simulink model "sim1"  (R2025a)
settings: Solver=VariableStepAuto  StartTime=0.0  StopTime=150  RelTol=1e-3
InitFcn:
  | clc;
  | close all;
  | clear;
  | s=tf('s');
  | G11=(0.806*s+0.264)/(s^2+1.15*s+0.202);
  | G12=-(15*s+1.42)/(s^3+12.8*s^2+13.6*s+2.36);
  | G21=(1.95*s^2+2.12*s+0.49)/(s^3+9.15*s^2+9.39*s+1.62);
  | G22=(7.14*s^2+25.8*s+9.35)/(s^4+20.8*s^3+116.4*s^2+111.6*s+18.8);
  | G=[G11,G12;G21,G22];
  | a11=[1 1.15 0.202];
  | a12=[1 12.8 13.6 2.36];
  | a21=[1 9.15 9.39 1.62];
  | a22=[1 20.8 116.4 111.6 18.8];
  | b11=[0.806 0.264];
  | b12=-[15 1.42];
  | b21=[1.95 2.12 0.49];
  | b22=[7.14 25.8 9.35];
  | K=[2,2.5;-6,5.5];
  | Q11=K(1,1)*G11+K(2,1)*G12;
  | Q12=K(1,2)*G11+K(2,2)*G12;
  | Q21=K(1,1)*G21+K(2,1)*G22;
  | Q22=K(1,2)*G21+K(2,2)*G22;
  | Q=[Q11,Q12;Q21,Q22];
  | % Gershgorinbands_MIMO(Q)
  | f1=1;
  | f2=1;
  | t11=(1/f1+Q11);
  | t12=(Q12);
  | t21=(Q21);
  | t22=(1/f2+Q22);
  | C1=pidtune(t11,'pi');
  | C2=pidtune(t22,'pi');
  | P1=C1.Kp;
  | I1=C1.Ki;
  | D1=C1.Kd;
  | P2=C2.Kp;
  | I2=C2.Ki;
  | D2=C2.Kd;
StopFcn:
  | close all;
  | subplot(1,2,1)
  | plot(out.tout,out.y_ref.data(:,1),'-.','LineWidth',3.5)
  | hold on
  | plot(out.tout,out.y.data(:,1),'LineWidth',2.5)
  | xlabel('time')
  | ylabel('y_1')
  | grid
  | subplot(1,2,2)
  | plot(out.tout,out.y_ref.data(:,2),'-.','LineWidth',3.5)
  | hold on
  | plot(out.tout,out.y.data(:,2),'LineWidth',2.5)
  | xlabel('time')
  | ylabel('y_2')
  | grid
  | sgtitle('System response')
  | 
  | figure()
  | subplot(1,2,1)
  | plot(out.tout,out.u.data(:,1),'LineWidth',2.5)
  | xlabel('time')
  | ylabel('u_1')
  | grid
  | subplot(1,2,2)
  | plot(out.tout,out.u.data(:,2),'LineWidth',2.5)
  | xlabel('time')
  | ylabel('u_2')
  | grid
  | sgtitle('Control Signal')
libraries: slpidlib x2, simulink x2
settings Model: Creator=rz97e  LastModifiedBy=sohrab
settings ModelReferenceCC: EnableRefExpFcnMdlSchedulingChecks=on
settings RTWCC: GPUComputeCapability=3.5

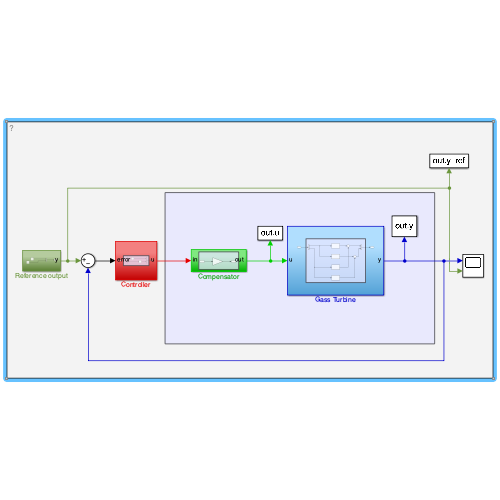
[thumbnail: Simulink's stored preview of the top-level diagram]
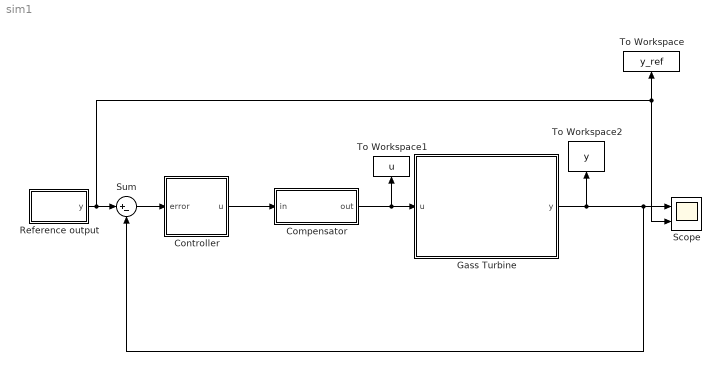
== system sim1 ==
  Compensator : Subsystem
  Controller : Subsystem
  Gass Turbine : Subsystem
  Reference output : Subsystem
  Scope : Scope  NumInputPorts=2
      settings: ActiveDisplayYMinimum=-0.55203  ActiveDisplayYMaximum=1.55201
  Sum : Sum  Inputs=|+-
  To Workspace : ToWorkspace  VariableName=y_ref  SaveFormat=Timeseries  SampleTime=-1
  To Workspace1 : ToWorkspace  VariableName=u  SaveFormat=Timeseries  SampleTime=-1
  To Workspace2 : ToWorkspace  VariableName=y  SaveFormat=Timeseries  SampleTime=-1
  wires:
  Gass Turbine/1(y) -> To Workspace2/1, Sum/2, Scope/1
  Reference output/1(y) -> Sum/1, To Workspace/1, Scope/2
  Compensator/1(out) -> To Workspace1/1, Gass Turbine/1(u)
  Controller/1(u) -> Compensator/1(in)
  Sum/1 -> Controller/1(error)

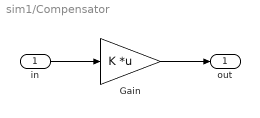
== system sim1/Compensator ==
  in : Inport
  Gain : Gain  Gain=K  Multiplication=Matrix(K*u) (u vector)
  out : Outport
  wires:
  in/1 -> Gain/1
  Gain/1 -> out/1

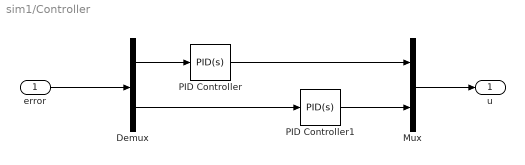
== system sim1/Controller ==
  error : Inport
  Demux : Demux  Outputs=2
  Mux : Mux  Inputs=2
  PID Controller : slpidlib/PID Controller  Controller=PID  Form=Parallel  TimeDomain=Continuous-time  UseExternalTs=off  SampleTime=-1  IntegratorMethod=Forward Euler  FilterMethod=Forward Euler  ControllerParametersSource=internal  P=P1  I=I1  UseKiTs=off  D=D1  UseExternalDerivativeSource=off  N=100  UseFilter=on  TunerSelectOption=Transfer Function Based (PID Tuner App)  InitialConditionSource=internal  InitialConditionForIntegrator=0  InitialConditionForFilter=0  DifferentiatorICPrevScaledInput=0  ExternalReset=none  TrackingMode=off  Kt=1  LimitOutput=off  SatLimitsSource=internal  UpperSaturationLimit=inf  LowerSaturationLimit=-inf  LinearizeAsGain=on  AntiWindupMode=none  Kb=1  LimitIntegrator=off  UpperIntegratorSaturationLimit=inf  LowerIntegratorSaturationLimit=-inf  POutMin=[]  POutMax=[]  IOutMin=[]  IOutMax=[]  DOutMin=[]  DOutMax=[]  NOutMin=[]  NOutMax=[]  SumOutMin=[]  SumOutMax=[]  SaturationOutMin=[]  SaturationOutMax=[]  PParamMin=[]  PParamMax=[]  IParamMin=[]  IParamMax=[]  DParamMin=[]  DParamMax=[]  NParamMin=[]  NParamMax=[]  KbParamMin=[]  KbParamMax=[]  KtParamMin=[]  KtParamMax=[]  KbOutMin=[]  KbOutMax=[]  KtOutMin=[]  KtOutMax=[]  IntegratorOutMin=[]  IntegratorOutMax=[]  FilterOutMin=[]  FilterOutMax=[]  SumI1OutMin=[]  SumI1OutMax=[]  SumI2OutMin=[]  SumI2OutMax=[]  SumI3OutMin=[]  SumI3OutMax=[]  SumI4OutMin=[]  SumI4OutMax=[]  SumDOutMin=[]  SumDOutMax=[]  DifferentiatorOutMin=[]  DifferentiatorOutMax=[]  FilterDiffOutCoefMin=[]  FilterDiffOutCoefMax=[]  ReciprocalOutMin=[]  ReciprocalOutMax=[]  SumDenOutMin=[]  SumDenOutMax=[]  SumNumOutMin=[]  SumNumOutMax=[]  DivideOutMin=[]  DivideOutMax=[]  UdiffTsProdOutMin=[]  UdiffTsProdOutMax=[]  NTsProdOutMin=[]  NTsProdOutMax=[]  UintegralTsProdOutMin=[]  UintegralTsProdOutMax=[]  UngainTsProdOutMin=[]  UngainTsProdOutMax=[]  ClampingZeroOutDataTypeStr=Inherit: Inherit via back propagation  ClampingZeroOutMin=[]  ClampingZeroOutMax=[]  FilterDenConstantOutDataTypeStr=Inherit: Inherit via back propagation  FilterDenConstantOutMin=[]  FilterDenConstantOutMax=[]  PCopyOutDataTypeStr=Inherit: Inherit via back propagation  PCopyOutMin=[]  PCopyOutMax=[]  NCopyOutDataTypeStr=Inherit: Inherit via back propagation  NCopyOutMin=[]  NCopyOutMax=[]  IntegratorContinuousStateAttributes=''  IntegratorStateMustResolveToSignalObject=off  IntegratorRTWStateStorageClass=Auto  FilterContinuousStateAttributes=''  FilterStateMustResolveToSignalObject=off  FilterRTWStateStorageClass=Auto  ParallelPVariant=InternalParameters  IdealPVariant=Disabled  IVariant=InternalParameters  DVariant=InternalParameters  IntegratorVariant=Continuous  SatVariant=Disabled  AWVariant=Passthrough  PCopyVariant=Disabled  TRVariant=Disabled  FdbkBlocksVariant=Forward  IdealPFdbkVariant=Disabled  SatFdbkVariant=Disabled  DerivativeFilterVariant=ContFilter  NVariant=InternalParameters  NCopyVariant=Disabled  FilterICVariant=InternalICsFilter  IntegratorICVariant=InternalICs  ExternalResetVariant=Disabled  TRSumVariant=Passthrough  SumFdbkVariant=Disabled  SumVariant=Sum_PID  TsampFilterVariant=InternalTs  TsampNgainVariant=Passthrough  TsampIntegralVariant=Disabled_SignalSpec  ExternalSaturationOutDataTypeStr=Inherit: Same as second input  DerivativeSourceVariant=ErrorSignal  PreIntVariant=InternalPreInt
  PID Controller1 : slpidlib/PID Controller  Controller=PID  Form=Parallel  TimeDomain=Continuous-time  UseExternalTs=off  SampleTime=-1  IntegratorMethod=Forward Euler  FilterMethod=Forward Euler  ControllerParametersSource=internal  P=P2  I=I2  UseKiTs=off  D=D2  UseExternalDerivativeSource=off  N=100  UseFilter=on  TunerSelectOption=Transfer Function Based (PID Tuner App)  InitialConditionSource=internal  InitialConditionForIntegrator=0  InitialConditionForFilter=0  DifferentiatorICPrevScaledInput=0  ExternalReset=none  TrackingMode=off  Kt=1  LimitOutput=off  SatLimitsSource=internal  UpperSaturationLimit=inf  LowerSaturationLimit=-inf  LinearizeAsGain=on  AntiWindupMode=none  Kb=1  LimitIntegrator=off  UpperIntegratorSaturationLimit=inf  LowerIntegratorSaturationLimit=-inf  POutMin=[]  POutMax=[]  IOutMin=[]  IOutMax=[]  DOutMin=[]  DOutMax=[]  NOutMin=[]  NOutMax=[]  SumOutMin=[]  SumOutMax=[]  SaturationOutMin=[]  SaturationOutMax=[]  PParamMin=[]  PParamMax=[]  IParamMin=[]  IParamMax=[]  DParamMin=[]  DParamMax=[]  NParamMin=[]  NParamMax=[]  KbParamMin=[]  KbParamMax=[]  KtParamMin=[]  KtParamMax=[]  KbOutMin=[]  KbOutMax=[]  KtOutMin=[]  KtOutMax=[]  IntegratorOutMin=[]  IntegratorOutMax=[]  FilterOutMin=[]  FilterOutMax=[]  SumI1OutMin=[]  SumI1OutMax=[]  SumI2OutMin=[]  SumI2OutMax=[]  SumI3OutMin=[]  SumI3OutMax=[]  SumI4OutMin=[]  SumI4OutMax=[]  SumDOutMin=[]  SumDOutMax=[]  DifferentiatorOutMin=[]  DifferentiatorOutMax=[]  FilterDiffOutCoefMin=[]  FilterDiffOutCoefMax=[]  ReciprocalOutMin=[]  ReciprocalOutMax=[]  SumDenOutMin=[]  SumDenOutMax=[]  SumNumOutMin=[]  SumNumOutMax=[]  DivideOutMin=[]  DivideOutMax=[]  UdiffTsProdOutMin=[]  UdiffTsProdOutMax=[]  NTsProdOutMin=[]  NTsProdOutMax=[]  UintegralTsProdOutMin=[]  UintegralTsProdOutMax=[]  UngainTsProdOutMin=[]  UngainTsProdOutMax=[]  ClampingZeroOutDataTypeStr=Inherit: Inherit via back propagation  ClampingZeroOutMin=[]  ClampingZeroOutMax=[]  FilterDenConstantOutDataTypeStr=Inherit: Inherit via back propagation  FilterDenConstantOutMin=[]  FilterDenConstantOutMax=[]  PCopyOutDataTypeStr=Inherit: Inherit via back propagation  PCopyOutMin=[]  PCopyOutMax=[]  NCopyOutDataTypeStr=Inherit: Inherit via back propagation  NCopyOutMin=[]  NCopyOutMax=[]  IntegratorContinuousStateAttributes=''  IntegratorStateMustResolveToSignalObject=off  IntegratorRTWStateStorageClass=Auto  FilterContinuousStateAttributes=''  FilterStateMustResolveToSignalObject=off  FilterRTWStateStorageClass=Auto  ParallelPVariant=InternalParameters  IdealPVariant=Disabled  IVariant=InternalParameters  DVariant=InternalParameters  IntegratorVariant=Continuous  SatVariant=Disabled  AWVariant=Passthrough  PCopyVariant=Disabled  TRVariant=Disabled  FdbkBlocksVariant=Forward  IdealPFdbkVariant=Disabled  SatFdbkVariant=Disabled  DerivativeFilterVariant=ContFilter  NVariant=InternalParameters  NCopyVariant=Disabled  FilterICVariant=InternalICsFilter  IntegratorICVariant=InternalICs  ExternalResetVariant=Disabled  TRSumVariant=Passthrough  SumFdbkVariant=Disabled  SumVariant=Sum_PID  TsampFilterVariant=InternalTs  TsampNgainVariant=Passthrough  TsampIntegralVariant=Disabled_SignalSpec  ExternalSaturationOutDataTypeStr=Inherit: Same as second input  DerivativeSourceVariant=ErrorSignal  PreIntVariant=InternalPreInt
  u : Outport
  wires:
  error/1 -> Demux/1
  Mux/1 -> u/1
  Demux/2 -> PID Controller1/1
  PID Controller1/1 -> Mux/2
  PID Controller/1 -> Mux/1
  Demux/1 -> PID Controller/1

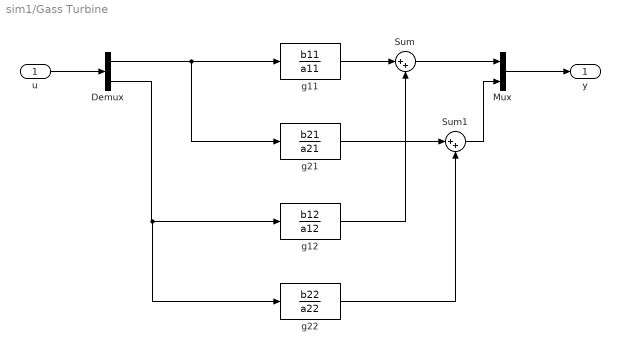
== system sim1/Gass Turbine ==
  u : Inport
  Demux : Demux  Outputs=2
  Mux : Mux  Inputs=2
  Sum : Sum  Inputs=|++
  Sum1 : Sum  Inputs=|++
  g11 : TransferFcn  Numerator=b11  Denominator=a11
  g12 : TransferFcn  Numerator=b12  Denominator=a12
  g21 : TransferFcn  Numerator=b21  Denominator=a21
  g22 : TransferFcn  Numerator=b22  Denominator=a22
  y : Outport
  wires:
  g11/1 -> Sum/1
  g12/1 -> Sum/2
  g21/1 -> Sum1/1
  g22/1 -> Sum1/2
  u/1 -> Demux/1
  Sum/1 -> Mux/1
  Sum1/1 -> Mux/2
  Mux/1 -> y/1
  Demux/1 -> g21/1, g11/1
  Demux/2 -> g22/1, g12/1

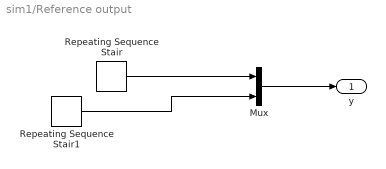
== system sim1/Reference output ==
  Mux : Mux  Inputs=2
  Repeating Sequence Stair : simulink/Sources/Repeating Sequence Stair  OutValues=[0 1 ].'  tsamp=40  OutMin=[]  OutMax=[]  OutDataTypeStr=double  OutputDataTypeScalingMode=double  OutDataType=fixdt(0,8)  ConRadixGroup=Best Precision: Vector-wise  OutScaling=2^-12
  Repeating Sequence Stair1 : simulink/Sources/Repeating Sequence Stair  OutValues=[1 1 1 0 0 0 1].'  tsamp=30  OutMin=[]  OutMax=[]  OutDataTypeStr=double  OutputDataTypeScalingMode=double  OutDataType=fixdt(0,8)  ConRadixGroup=Best Precision: Vector-wise  OutScaling=2^-12
  y : Outport
  wires:
  Mux/1 -> y/1
  Repeating Sequence Stair/1 -> Mux/1
  Repeating Sequence Stair1/1 -> Mux/2
